simulink model "sl_subsys_fcncall9"  (Simulink 6.0)
settings: Solver=FixedStepDiscrete  StartTime=0.0  StopTime=10.0  FixedStep=0.1  RelTol=1e-3
undefined symbols (not defined in the file or in its folder): DiscIntNeverNeededParam
settings Model: CovMetricSettings=d  Creator=The MathWorks Inc.  LastModifiedBy=batserve  ExtModeAutoUpdateStatusClock=off
settings DataIOCC: SignalLoggingName=logsOut
settings OptimizationCC: BlockReduction=off  BooleanDataType=off  OptimizeModelRefInitCode=on  LifeSpan=1
settings DebuggingCC: CheckExecutionContextPreStartOutputMsg=on  CheckExecutionContextRuntimeOutputMsg=on  SolverPrmCheckMsg=none
settings ModelReferenceCC: UpdateModelReferenceTargets=IfOutOfDate
settings RTWCC: SystemTargetFile=ert.tlc  TemplateMakefile=ert_default_tmf  Description=RTW Embedded Coder (no auto configuration)  GenerateReport=on  ProcessScript=ert_make_rtw_hook  IncludeHyperlinkInReport=on  LaunchReport=on
settings CodeAppCC: IgnoreCustomStorageClasses=off
settings ERTTargetCC: TargetFcnLib=ansi_tfl_tmw.mat  GenFloatMathFcnCalls=ANSI_C  GenerateSampleERTMain=on  SupportContinuousTime=on  SupportNonInlinedSFcns=on  RootIOFormat=Individual Arguments  ERTCustomFileTemplate=example_file_process.tlc  InitialValueSource=Model

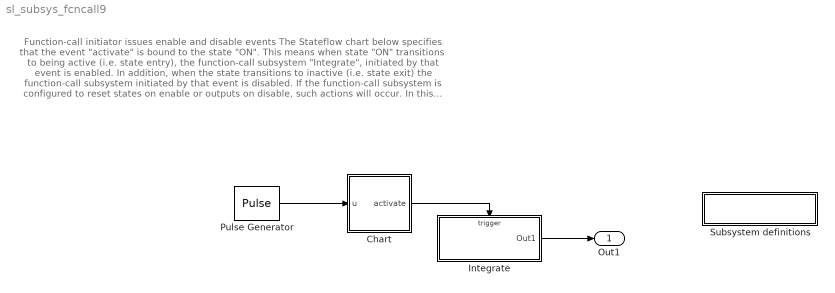
== system sl_subsys_fcncall9 ==
  note: Function-call initiator issues enable and disable events
      |
      | The Stateflow chart below specifies that the event "activate" is bound to the state
      | "ON".  This means when state "ON" transitions to being active (i.e. state entry),
      | the function-call subsystem "Integrate", initiated by that event is enabled. In
      | addition, when the state transitions to inactive (i.e. state exit) the
      | function-call subsystem initiated by that event is disabled.  If the function-call
      | subsystem is configured to reset states on enable or outputs on disable, such actions
      | will occur.  In this example the subsystem does in fact request that its states and
      | outputs be reset upon enable and disable, respectively.
  " Subsystem definitions" : Subsystem  PropExecContextAcrossSSBoundary=on
      settings: OpenFcn=helpview([matlabroot,'/toolbox/simulink/simdemos/sl_subsys_definitions.html']);
      mask Display: disp('Subsystem\ndefinitions')
  Chart : Stateflow chart  PropExecContextAcrossSSBoundary=on
  Integrate : Subsystem  TreatAsAtomicUnit=on  PropExecContextAcrossSSBoundary=on
  Pulse Generator : DiscretePulseGenerator  Period=20  PulseWidth=10  PhaseDelay=10  SampleTime=0.1
  Out1 : Outport
  wires:
  Integrate/1(Out1) -> Out1/1
  Chart/1(activate) -> Integrate/Trigger
  Pulse Generator/1 -> Chart/1(u)

== system sl_subsys_fcncall9/ Subsystem definitions ==

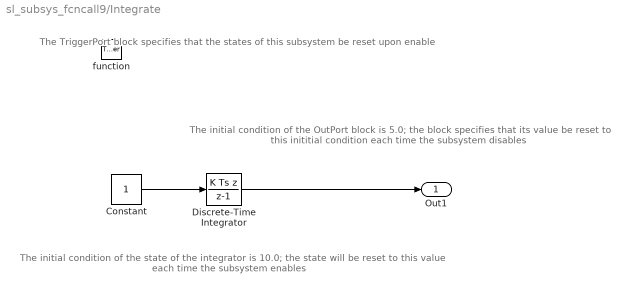
== system sl_subsys_fcncall9/Integrate ==
  note: The TriggerPort block specifies that the
      | states of this subsystem be reset
      | upon enable
  note: The initial condition of the state of the integrator
      | is 10.0; the state will be reset to this value each
      | time the subsystem enables
  note: The initial condition of the OutPort block
      | is 5.0; the block specifies that its value be
      | reset to this inititial condition each time the
      | subsystem disables
  function : TriggerPort  TriggerType=function-call  StatesWhenEnabling=reset  SampleTime=-1
  Constant : Constant
  Discrete-Time Integrator : DiscreteIntegrator  IntegratorMethod=Integration: Backward Euler  InitialCondition=10  SampleTime=-1  ICPrevOutput=DiscIntNeverNeededParam  ICPrevScaledInput=DiscIntNeverNeededParam
  Out1 : Outport  OutputWhenDisabled=reset  InitialOutput=5
  wires:
  Constant/1 -> Discrete-Time Integrator/1
  Discrete-Time Integrator/1 -> Out1/1

== stateflow chart Chart ==
  state OFF
  state ON/
    bind: activate
    (junction 5) -> (junction 6) : {activate;}
    (default) -> (junction 5)
    ON -> (junction 5)
  OFF -> ON : [u > 0]
  ON -> OFF : [u < 1]
  (default) -> OFF
  data: u input double
  events: activate output FUNCTION_CALL_EVENT
